simulink model "Senior_Capstone_Model"  (R2022b)
settings: Solver=VariableStepAuto  StartTime=0.0  StopTime=100  RelTol=1e-3
undefined symbols (not defined in the file): A, C_D, C_L, g, i_0, i_x, m, Mu, r, rho
libraries: simulink x1
settings Model: Creator=amayk  LastModifiedBy=amayk

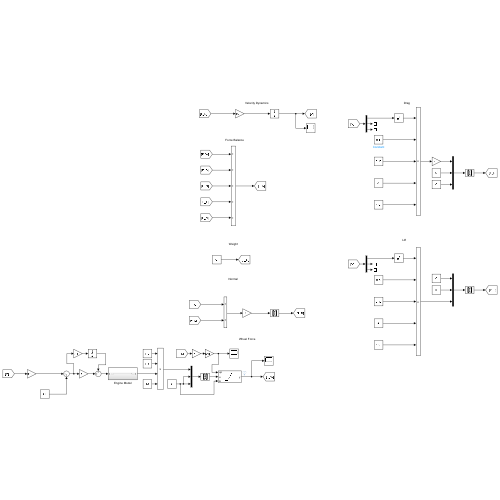
[thumbnail: Simulink's stored preview of the top-level diagram]
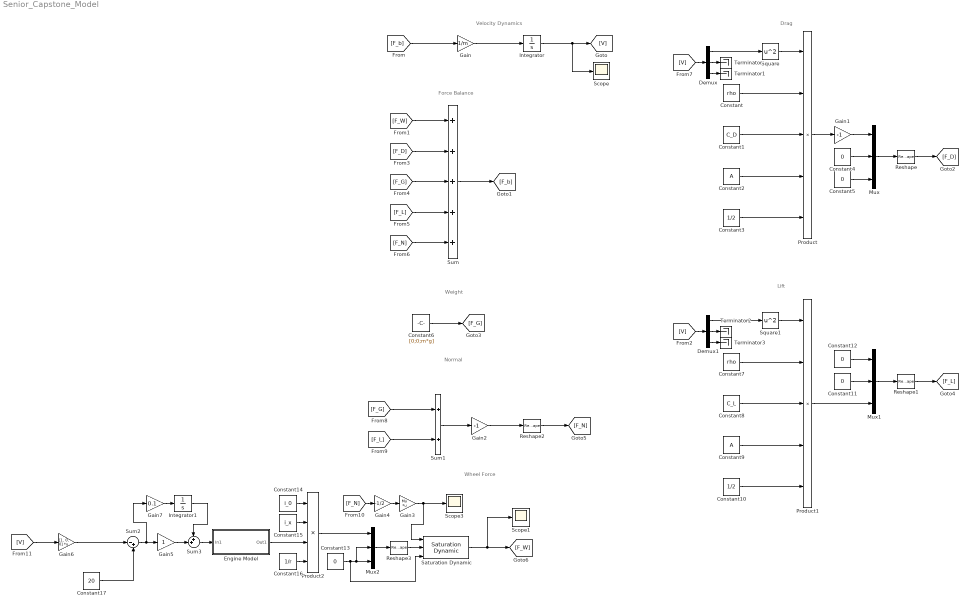
== system Senior_Capstone_Model ==
  note: Wheel Force
  note: Normal
  note: Lift
  note: Weight
  note: Drag
  note: Force Balance
  note: Velocity Dynamics
  Constant : Constant  Value=rho
  Constant1 : Constant  Value=C_D
  Constant10 : Constant  Value=1/2
  Constant{4..5,11..13} (5 alike) : Constant  Value=0
  Constant14 : Constant  Value=i_0
  Constant15 : Constant  Value=i_x
  Constant16 : Constant  Value=1/r
  Constant17 : Constant  Value=20
  Constant2 : Constant  Value=A
  Constant3 : Constant  Value=1/2
  Constant6 : Constant  Value=[0;0;m*g]
  Constant7 : Constant  Value=rho
  Constant8 : Constant  Value=C_L
  Constant9 : Constant  Value=A
  Demux : Demux  Outputs=3
  Demux1 : Demux  Outputs=3
  Engine Model : Subsystem
  Gain : Gain  Gain=1/m
  Gain1 : Gain  Gain=-1
  Gain2 : Gain  Gain=-1
  Gain3 : Gain  Gain=Mu  Multiplication=Matrix(K*u)
  Gain4 : Gain  Gain=-1/2
  Gain5 : Gain
  Gain6 : Gain  Gain=[1, 0, 0]  Multiplication=Matrix(K*u)
  Gain7 : Gain  Gain=0.1
  Integrator : Integrator
  Integrator1 : Integrator
  Mux : Mux  Inputs=3
  Mux1 : Mux  Inputs=3
  Mux2 : Mux  Inputs=3
  Product : Product  Inputs=5
  Product1 : Product  Inputs=5
  Product2 : Product  Inputs=4
  Reshape{,1..3} (4 alike) : Reshape  OutputDimensionality=Column vector (2-D)
  Saturation Dynamic : simulink/Discontinuities/Saturation Dynamic  OutMin=[]  OutMax=[]  OutDataTypeStr=Inherit: Same as second input  OutDataType=fixdt(1, 16)  OutScaling=2^-10  DoSatur=off
  Scope : Scope
  Scope1 : Scope
  Scope3 : Scope
  Square : Math  Operator=square
  Square1 : Math  Operator=square
  Sum : Sum  Inputs=+++++
  Sum1 : Sum
  Sum2 : Sum  Inputs=|-+
  Sum3 : Sum  Inputs=++|
  Terminator{,1..3} (4 alike) : Terminator
  wires:
  [F_b] -> Gain/1
  Gain/1 -> Integrator/1
  Integrator/1 -> Scope/1, [V]
  [F_W] -> Sum/1
  Sum/1 -> [F_b]
  Square/1 -> Product/1
  Constant/1 -> Product/2
  Constant1/1 -> Product/3
  Constant2/1 -> Product/4
  Constant3/1 -> Product/5
  Product/1 -> Gain1/1
  [V] -> Demux/1
  Demux/1 -> Square/1
  Demux/2 -> Terminator/1
  Demux/3 -> Terminator1/1
  Gain1/1 -> Mux/1
  Constant4/1 -> Mux/2
  Constant5/1 -> Mux/3
  Mux/1 -> Reshape/1
  Reshape/1 -> [F_D]
  [F_D] -> Sum/2
  [F_G] -> Sum/3
  [F_L] -> Sum/4
  [F_N] -> Sum/5
  Constant6/1 -> [F_G]
  Constant11/1 -> Mux1/2
  Mux1/1 -> Reshape1/1
  Demux1/1 -> Square1/1
  Constant12/1 -> Mux1/1
  [V] -> Demux1/1
  Demux1/3 -> Terminator3/1
  Constant8/1 -> Product1/3
  Constant9/1 -> Product1/4
  Constant10/1 -> Product1/5
  Square1/1 -> Product1/1
  Reshape1/1 -> [F_L]
  Demux1/2 -> Terminator2/1
  Constant7/1 -> Product1/2
  Product1/1 -> Mux1/3
  [F_G] -> Sum1/1
  [F_L] -> Sum1/2
  Sum1/1 -> Gain2/1
  Gain2/1 -> Reshape2/1
  Reshape2/1 -> [F_N]
  Constant13/1 -> Saturation Dynamic/3, Mux2/2, Mux2/3
  Constant14/1 -> Product2/1
  Constant15/1 -> Product2/2
  Engine Model/1(Out1) -> Product2/3
  Constant16/1 -> Product2/4
  [F_N] -> Gain4/1
  Gain3/1 -> Saturation Dynamic/1, Scope3/1
  Mux2/1 -> Reshape3/1
  Product2/1 -> Mux2/1
  Gain4/1 -> Gain3/1
  Reshape3/1 -> Saturation Dynamic/2
  Saturation Dynamic/1 -> Scope1/1, [F_W]
  Gain6/1 -> Sum2/1
  Constant17/1 -> Sum2/2
  Sum2/1 -> Gain7/1, Gain5/1
  [V] -> Gain6/1
  Integrator1/1 -> Sum3/1
  Sum3/1 -> Engine Model/1(In1)
  Gain5/1 -> Sum3/2
  Gain7/1 -> Integrator1/1

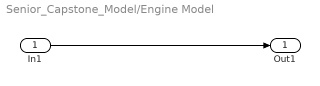
== system Senior_Capstone_Model/Engine Model ==
  In1 : Inport
  Out1 : Outport
  wires:
  In1/1 -> Out1/1
